simulink model "TopLevelModel"  (R2023a)
settings: Solver=VariableStepAuto  StartTime=0.0  StopTime=inf  RelTol=1e-3
values from neighbouring files (symbols this model uses):
  b = 40.6518    [TopLevelModelParameters.m]
  B1 = 0.0042    [TopLevelModelParameters.m]
  B2 = 0.0084    [TopLevelModelParameters.m]
  J1 = 7e-5    (= 7e-05)    [TopLevelModelParameters.m]
  J2 = 8e-5    (= 8e-05)    [TopLevelModelParameters.m]
  k1 = 2.6552e5    (= 265520)    [TopLevelModelParameters.m]
  k2 = 2.6552e5    (= 265520)    [TopLevelModelParameters.m]
  k3 = 11.777e4    (= 117770)    [TopLevelModelParameters.m]
  Kb = 23e-3    (= 0.023)    [TopLevelModelParameters.m]
  Kt = 23e-3    (= 0.023)    [TopLevelModelParameters.m]
  L = 0.1    [TopLevelModelParameters.m]
  m = 2    [TopLevelModelParameters.m]
  R = 0.71    [TopLevelModelParameters.m]
  r = 0.0194    [TopLevelModelParameters.m]
undefined symbols (not defined in the file or in its folder): J, Kd, Ke
libraries: fl_lib x40, fl_ps_legacy_lib x16, nesl_utility x12, slpidlib x10, SignalEditorBlockLib x4, ee_lib x4, simulink x2
(part 2 of 3)

== system TopLevelModel/Belt7 ==
  V1 : Inport
  Constant3 : Constant  Commented=on  Value=0.2
  Constant4 : Constant  Commented=on  Value=0
  PID Controller1 : slpidlib/PID Controller  Commented=on  Controller=PID  Form=Parallel  TimeDomain=Continuous-time  UseExternalTs=off  SampleTime=-1  IntegratorMethod=Forward Euler  FilterMethod=Forward Euler  ControllerParametersSource=internal  P=29.8496571480823  I=152.933850283855  UseKiTs=off  D=-0.451147774638306  N=4.48716691500189  UseFilter=on  TunerSelectOption=Transfer Function Based (PID Tuner App)  InitialConditionSource=internal  InitialConditionForIntegrator=0  InitialConditionForFilter=0  DifferentiatorICPrevScaledInput=0  ExternalReset=none  TrackingMode=off  Kt=1  LimitOutput=off  SatLimitsSource=internal  UpperSaturationLimit=inf  LowerSaturationLimit=-inf  LinearizeAsGain=on  AntiWindupMode=none  Kb=1  LimitIntegrator=off  UpperIntegratorSaturationLimit=inf  LowerIntegratorSaturationLimit=-inf  POutMin=[]  POutMax=[]  IOutMin=[]  IOutMax=[]  DOutMin=[]  DOutMax=[]  NOutMin=[]  NOutMax=[]  SumOutMin=[]  SumOutMax=[]  SaturationOutMin=[]  SaturationOutMax=[]  PParamMin=[]  PParamMax=[]  IParamMin=[]  IParamMax=[]  DParamMin=[]  DParamMax=[]  NParamMin=[]  NParamMax=[]  KbParamMin=[]  KbParamMax=[]  KtParamMin=[]  KtParamMax=[]  KbOutMin=[]  KbOutMax=[]  KtOutMin=[]  KtOutMax=[]  IntegratorOutMin=[]  IntegratorOutMax=[]  FilterOutMin=[]  FilterOutMax=[]  SumI1OutMin=[]  SumI1OutMax=[]  SumI2OutMin=[]  SumI2OutMax=[]  SumI3OutMin=[]  SumI3OutMax=[]  SumI4OutMin=[]  SumI4OutMax=[]  SumDOutMin=[]  SumDOutMax=[]  DifferentiatorOutMin=[]  DifferentiatorOutMax=[]  FilterDiffOutCoefMin=[]  FilterDiffOutCoefMax=[]  ReciprocalOutMin=[]  ReciprocalOutMax=[]  SumDenOutMin=[]  SumDenOutMax=[]  SumNumOutMin=[]  SumNumOutMax=[]  DivideOutMin=[]  DivideOutMax=[]  UdiffTsProdOutMin=[]  UdiffTsProdOutMax=[]  NTsProdOutMin=[]  NTsProdOutMax=[]  UintegralTsProdOutMin=[]  UintegralTsProdOutMax=[]  UngainTsProdOutMin=[]  UngainTsProdOutMax=[]  ClampingZeroOutDataTypeStr=Inherit: Inherit via back propagation  ClampingZeroOutMin=[]  ClampingZeroOutMax=[]  FilterDenConstantOutDataTypeStr=Inherit: Inherit via back propagation  FilterDenConstantOutMin=[]  FilterDenConstantOutMax=[]  PCopyOutDataTypeStr=Inherit: Inherit via back propagation  PCopyOutMin=[]  PCopyOutMax=[]  NCopyOutDataTypeStr=Inherit: Inherit via back propagation  NCopyOutMin=[]  NCopyOutMax=[]  IntegratorContinuousStateAttributes=''  IntegratorStateMustResolveToSignalObject=off  IntegratorRTWStateStorageClass=Auto  FilterContinuousStateAttributes=''  FilterStateMustResolveToSignalObject=off  FilterRTWStateStorageClass=Auto  ParallelPVariant=InternalParameters  IdealPVariant=Disabled  IVariant=InternalParameters  DVariant=InternalParameters  IntegratorVariant=Continuous  SatVariant=Disabled  AWVariant=Passthrough  PCopyVariant=Disabled  TRVariant=Disabled  FdbkBlocksVariant=Forward  IdealPFdbkVariant=Disabled  SatFdbkVariant=Disabled  DerivativeFilterVariant=ContFilter  NVariant=InternalParameters  NCopyVariant=Disabled  FilterICVariant=InternalICsFilter  IntegratorICVariant=InternalICs  ExternalResetVariant=Disabled  TRSumVariant=Passthrough  SumFdbkVariant=Disabled  SumVariant=Sum_PID  TsampFilterVariant=InternalTs  TsampNgainVariant=Passthrough  TsampIntegralVariant=Disabled_SignalSpec  ExternalSaturationOutDataTypeStr=Inherit: Same as second input
  Subsystem2 : Subsystem  Commented=on
  Sum1 : Sum  Commented=on  Inputs=|+-
  Switch1 : Switch  Commented=on  Criteria=u2 ~= 0  Threshold=1  SaturateOnIntegerOverflow=off  InputSameDT=off
  drive pulley velocity : Outport
  load velocity : Outport  Port=2
  load position : Outport  Port=3
  driven pulley Velocity : Outport  Port=4
  wires:
  Switch1/1 -> Sum1/1
  Sum1/1 -> PID Controller1/1
  V1/1 -> Switch1/2
  Subsystem2/2(load velocity) -> load velocity/1, Sum1/2  "Velocity"
  Constant3/1 -> Switch1/1
  Constant4/1 -> Switch1/3
  PID Controller1/1 -> Subsystem2/1(Voltage)
  Subsystem2/3(load position) -> load position/1
  Subsystem2/4(driven pulley Velocity) -> driven pulley Velocity/1
  Subsystem2/1(drive pulley velocity) -> drive pulley velocity/1

== system TopLevelModel/Belt8 ==
  V1 : Inport
  Constant3 : Constant  Commented=on  Value=0.2
  Constant4 : Constant  Commented=on  Value=0
  PID Controller1 : slpidlib/PID Controller  Commented=on  Controller=PID  Form=Parallel  TimeDomain=Continuous-time  UseExternalTs=off  SampleTime=-1  IntegratorMethod=Forward Euler  FilterMethod=Forward Euler  ControllerParametersSource=internal  P=29.8496571480823  I=152.933850283855  UseKiTs=off  D=-0.451147774638306  N=4.48716691500189  UseFilter=on  TunerSelectOption=Transfer Function Based (PID Tuner App)  InitialConditionSource=internal  InitialConditionForIntegrator=0  InitialConditionForFilter=0  DifferentiatorICPrevScaledInput=0  ExternalReset=none  TrackingMode=off  Kt=1  LimitOutput=off  SatLimitsSource=internal  UpperSaturationLimit=inf  LowerSaturationLimit=-inf  LinearizeAsGain=on  AntiWindupMode=none  Kb=1  LimitIntegrator=off  UpperIntegratorSaturationLimit=inf  LowerIntegratorSaturationLimit=-inf  POutMin=[]  POutMax=[]  IOutMin=[]  IOutMax=[]  DOutMin=[]  DOutMax=[]  NOutMin=[]  NOutMax=[]  SumOutMin=[]  SumOutMax=[]  SaturationOutMin=[]  SaturationOutMax=[]  PParamMin=[]  PParamMax=[]  IParamMin=[]  IParamMax=[]  DParamMin=[]  DParamMax=[]  NParamMin=[]  NParamMax=[]  KbParamMin=[]  KbParamMax=[]  KtParamMin=[]  KtParamMax=[]  KbOutMin=[]  KbOutMax=[]  KtOutMin=[]  KtOutMax=[]  IntegratorOutMin=[]  IntegratorOutMax=[]  FilterOutMin=[]  FilterOutMax=[]  SumI1OutMin=[]  SumI1OutMax=[]  SumI2OutMin=[]  SumI2OutMax=[]  SumI3OutMin=[]  SumI3OutMax=[]  SumI4OutMin=[]  SumI4OutMax=[]  SumDOutMin=[]  SumDOutMax=[]  DifferentiatorOutMin=[]  DifferentiatorOutMax=[]  FilterDiffOutCoefMin=[]  FilterDiffOutCoefMax=[]  ReciprocalOutMin=[]  ReciprocalOutMax=[]  SumDenOutMin=[]  SumDenOutMax=[]  SumNumOutMin=[]  SumNumOutMax=[]  DivideOutMin=[]  DivideOutMax=[]  UdiffTsProdOutMin=[]  UdiffTsProdOutMax=[]  NTsProdOutMin=[]  NTsProdOutMax=[]  UintegralTsProdOutMin=[]  UintegralTsProdOutMax=[]  UngainTsProdOutMin=[]  UngainTsProdOutMax=[]  ClampingZeroOutDataTypeStr=Inherit: Inherit via back propagation  ClampingZeroOutMin=[]  ClampingZeroOutMax=[]  FilterDenConstantOutDataTypeStr=Inherit: Inherit via back propagation  FilterDenConstantOutMin=[]  FilterDenConstantOutMax=[]  PCopyOutDataTypeStr=Inherit: Inherit via back propagation  PCopyOutMin=[]  PCopyOutMax=[]  NCopyOutDataTypeStr=Inherit: Inherit via back propagation  NCopyOutMin=[]  NCopyOutMax=[]  IntegratorContinuousStateAttributes=''  IntegratorStateMustResolveToSignalObject=off  IntegratorRTWStateStorageClass=Auto  FilterContinuousStateAttributes=''  FilterStateMustResolveToSignalObject=off  FilterRTWStateStorageClass=Auto  ParallelPVariant=InternalParameters  IdealPVariant=Disabled  IVariant=InternalParameters  DVariant=InternalParameters  IntegratorVariant=Continuous  SatVariant=Disabled  AWVariant=Passthrough  PCopyVariant=Disabled  TRVariant=Disabled  FdbkBlocksVariant=Forward  IdealPFdbkVariant=Disabled  SatFdbkVariant=Disabled  DerivativeFilterVariant=ContFilter  NVariant=InternalParameters  NCopyVariant=Disabled  FilterICVariant=InternalICsFilter  IntegratorICVariant=InternalICs  ExternalResetVariant=Disabled  TRSumVariant=Passthrough  SumFdbkVariant=Disabled  SumVariant=Sum_PID  TsampFilterVariant=InternalTs  TsampNgainVariant=Passthrough  TsampIntegralVariant=Disabled_SignalSpec  ExternalSaturationOutDataTypeStr=Inherit: Same as second input
  Subsystem2 : Subsystem  Commented=on
  Sum1 : Sum  Commented=on  Inputs=|+-
  Switch1 : Switch  Commented=on  Criteria=u2 ~= 0  Threshold=1  SaturateOnIntegerOverflow=off  InputSameDT=off
  drive pulley velocity : Outport
  load velocity : Outport  Port=2
  load position : Outport  Port=3
  driven pulley Velocity : Outport  Port=4
  wires:
  Switch1/1 -> Sum1/1
  Sum1/1 -> PID Controller1/1
  V1/1 -> Switch1/2
  Subsystem2/2(load velocity) -> load velocity/1, Sum1/2  "Velocity"
  Constant3/1 -> Switch1/1
  Constant4/1 -> Switch1/3
  PID Controller1/1 -> Subsystem2/1(Voltage)
  Subsystem2/3(load position) -> load position/1
  Subsystem2/4(driven pulley Velocity) -> driven pulley Velocity/1
  Subsystem2/1(drive pulley velocity) -> drive pulley velocity/1

== system TopLevelModel/Belt9 ==
  V1 : Inport
  Constant3 : Constant  Commented=on  Value=0.2
  Constant4 : Constant  Commented=on  Value=0
  PID Controller1 : slpidlib/PID Controller  Commented=on  Controller=PID  Form=Parallel  TimeDomain=Continuous-time  UseExternalTs=off  SampleTime=-1  IntegratorMethod=Forward Euler  FilterMethod=Forward Euler  ControllerParametersSource=internal  P=29.8496571480823  I=152.933850283855  UseKiTs=off  D=-0.451147774638306  N=4.48716691500189  UseFilter=on  TunerSelectOption=Transfer Function Based (PID Tuner App)  InitialConditionSource=internal  InitialConditionForIntegrator=0  InitialConditionForFilter=0  DifferentiatorICPrevScaledInput=0  ExternalReset=none  TrackingMode=off  Kt=1  LimitOutput=off  SatLimitsSource=internal  UpperSaturationLimit=inf  LowerSaturationLimit=-inf  LinearizeAsGain=on  AntiWindupMode=none  Kb=1  LimitIntegrator=off  UpperIntegratorSaturationLimit=inf  LowerIntegratorSaturationLimit=-inf  POutMin=[]  POutMax=[]  IOutMin=[]  IOutMax=[]  DOutMin=[]  DOutMax=[]  NOutMin=[]  NOutMax=[]  SumOutMin=[]  SumOutMax=[]  SaturationOutMin=[]  SaturationOutMax=[]  PParamMin=[]  PParamMax=[]  IParamMin=[]  IParamMax=[]  DParamMin=[]  DParamMax=[]  NParamMin=[]  NParamMax=[]  KbParamMin=[]  KbParamMax=[]  KtParamMin=[]  KtParamMax=[]  KbOutMin=[]  KbOutMax=[]  KtOutMin=[]  KtOutMax=[]  IntegratorOutMin=[]  IntegratorOutMax=[]  FilterOutMin=[]  FilterOutMax=[]  SumI1OutMin=[]  SumI1OutMax=[]  SumI2OutMin=[]  SumI2OutMax=[]  SumI3OutMin=[]  SumI3OutMax=[]  SumI4OutMin=[]  SumI4OutMax=[]  SumDOutMin=[]  SumDOutMax=[]  DifferentiatorOutMin=[]  DifferentiatorOutMax=[]  FilterDiffOutCoefMin=[]  FilterDiffOutCoefMax=[]  ReciprocalOutMin=[]  ReciprocalOutMax=[]  SumDenOutMin=[]  SumDenOutMax=[]  SumNumOutMin=[]  SumNumOutMax=[]  DivideOutMin=[]  DivideOutMax=[]  UdiffTsProdOutMin=[]  UdiffTsProdOutMax=[]  NTsProdOutMin=[]  NTsProdOutMax=[]  UintegralTsProdOutMin=[]  UintegralTsProdOutMax=[]  UngainTsProdOutMin=[]  UngainTsProdOutMax=[]  ClampingZeroOutDataTypeStr=Inherit: Inherit via back propagation  ClampingZeroOutMin=[]  ClampingZeroOutMax=[]  FilterDenConstantOutDataTypeStr=Inherit: Inherit via back propagation  FilterDenConstantOutMin=[]  FilterDenConstantOutMax=[]  PCopyOutDataTypeStr=Inherit: Inherit via back propagation  PCopyOutMin=[]  PCopyOutMax=[]  NCopyOutDataTypeStr=Inherit: Inherit via back propagation  NCopyOutMin=[]  NCopyOutMax=[]  IntegratorContinuousStateAttributes=''  IntegratorStateMustResolveToSignalObject=off  IntegratorRTWStateStorageClass=Auto  FilterContinuousStateAttributes=''  FilterStateMustResolveToSignalObject=off  FilterRTWStateStorageClass=Auto  ParallelPVariant=InternalParameters  IdealPVariant=Disabled  IVariant=InternalParameters  DVariant=InternalParameters  IntegratorVariant=Continuous  SatVariant=Disabled  AWVariant=Passthrough  PCopyVariant=Disabled  TRVariant=Disabled  FdbkBlocksVariant=Forward  IdealPFdbkVariant=Disabled  SatFdbkVariant=Disabled  DerivativeFilterVariant=ContFilter  NVariant=InternalParameters  NCopyVariant=Disabled  FilterICVariant=InternalICsFilter  IntegratorICVariant=InternalICs  ExternalResetVariant=Disabled  TRSumVariant=Passthrough  SumFdbkVariant=Disabled  SumVariant=Sum_PID  TsampFilterVariant=InternalTs  TsampNgainVariant=Passthrough  TsampIntegralVariant=Disabled_SignalSpec  ExternalSaturationOutDataTypeStr=Inherit: Same as second input
  Subsystem2 : Subsystem  Commented=on
  Sum1 : Sum  Commented=on  Inputs=|+-
  Switch1 : Switch  Commented=on  Criteria=u2 ~= 0  Threshold=1  SaturateOnIntegerOverflow=off  InputSameDT=off
  drive pulley velocity : Outport
  load velocity : Outport  Port=2
  load position : Outport  Port=3
  driven pulley Velocity : Outport  Port=4
  wires:
  Switch1/1 -> Sum1/1
  Sum1/1 -> PID Controller1/1
  V1/1 -> Switch1/2
  Subsystem2/2(load velocity) -> load velocity/1, Sum1/2  "Velocity"
  Constant3/1 -> Switch1/1
  Constant4/1 -> Switch1/3
  PID Controller1/1 -> Subsystem2/1(Voltage)
  Subsystem2/3(load position) -> load position/1
  Subsystem2/4(driven pulley Velocity) -> driven pulley Velocity/1
  Subsystem2/1(drive pulley velocity) -> drive pulley velocity/1

== system TopLevelModel/Controller ==
  Ref : Inport
  Position : Subsystem  VariantControl=Position
  Speed : Subsystem  VariantControl=Speed
  PWM : PMIOPort  Side=Right
  0v : PMIOPort  Port=2  Side=Right
  REV : PMIOPort  Port=3  Side=Right

== system TopLevelModel/Controller1 ==
  Ref : Inport
  Position : Subsystem  VariantControl=Position
  Speed : Subsystem  VariantControl=Speed
  PWM : PMIOPort  Side=Right
  0v : PMIOPort  Port=2  Side=Right
  REV : PMIOPort  Port=3  Side=Right

== system TopLevelModel/DC Motor10 ==
  note: Armature Controlled DC Motor
      |
      | $E_a = R_a \cdot I_a + L_a \cdot \frac{di_a}{dt} + K_b \cdot \frac{d\theta}{dt}$
      | $T_{m} = K_{t} \cdot I_{a}$
  Voltage : Inport
  Velocity : Inport  Port=2
  Constant1 : Constant  Value=R
  Gain1 : Gain  Gain=Kb
  Gain2 : Gain  Gain=1/L
  Gain3 : Gain  Gain=Kt
  Integrator : Integrator
  Product : Product
  Subtract : Sum  Inputs=+--
  Tourque : Outport
  wires:
  Voltage/1 -> Subtract/1
  Integrator/1 -> Product/1, Gain3/1  "i"
  Gain3/1 -> Tourque/1
  Gain1/1 -> Subtract/2
  Velocity/1 -> Gain1/1
  Constant1/1 -> Product/2
  Product/1 -> Subtract/3
  Gain2/1 -> Integrator/1  "i_dot"
  Subtract/1 -> Gain2/1

== system TopLevelModel/Sensing Angle ==
  MRRef : fl_lib/Mechanical/Rotational Elements/Mechanical Rotational Reference
  Motion Sensor : fl_lib/Mechanical/Mechanical Sensors/Ideal Rotational Motion Sensor  reference=foundation.enum.MeasurementReference.difference  acceleration_port=false  velocity_port=true  position_port=true  wrap_angle=simscape.enum.onoff.off  offset=0 rad
  deg : nesl_utility/PS-Simulink Converter  PhysicalDomain=network_engine_domain  SubClassName=ps_output  LeftPortType=input  RightPortType=output  PseudoPeriodic=off  Frequencies=[]  VectorFormat=1-D array  Unit=deg  AffineConversion=off
  R : PMIOPort  Side=Left
  theta : Outport  VectorParamsAs1DForOutWhenUnconnected=off
  wires:
  deg/1 -> theta/1
  connections:
  R/RConn1 -- Motion Sensor/LConn1
  Motion Sensor/RConn3 -- deg/LConn1
  MRRef/LConn1 -- Motion Sensor/RConn1

== system TopLevelModel/Sensing Angle1 ==
  MRRef : fl_lib/Mechanical/Rotational Elements/Mechanical Rotational Reference
  Motion Sensor : fl_lib/Mechanical/Mechanical Sensors/Ideal Rotational Motion Sensor  reference=foundation.enum.MeasurementReference.difference  acceleration_port=false  velocity_port=true  position_port=true  wrap_angle=simscape.enum.onoff.off  offset=0 rad
  deg : nesl_utility/PS-Simulink Converter  PhysicalDomain=network_engine_domain  SubClassName=ps_output  LeftPortType=input  RightPortType=output  PseudoPeriodic=off  Frequencies=[]  VectorFormat=1-D array  Unit=deg  AffineConversion=off
  R : PMIOPort  Side=Left
  theta : Outport  VectorParamsAs1DForOutWhenUnconnected=off
  wires:
  deg/1 -> theta/1
  connections:
  R/RConn1 -- Motion Sensor/LConn1
  Motion Sensor/RConn3 -- deg/LConn1
  MRRef/LConn1 -- Motion Sensor/RConn1

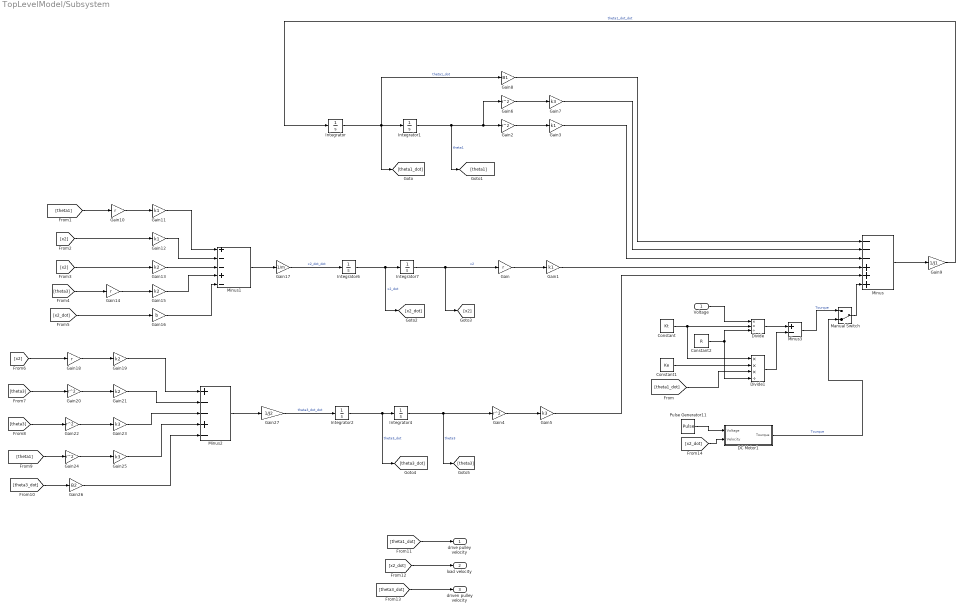
== system TopLevelModel/Subsystem ==
  Voltage : Inport
  Constant : Constant  Value=Kt
  Constant1 : Constant  Value=Ke
  Constant2 : Constant  Value=R
  DC Motor1 : Subsystem
  Divide : Product  Inputs=**/
  Divide1 : Product  Inputs=***/
  Gain{,10,14,18} (4 alike) : Gain  Gain=r
  Gain{1,3,11..12} (4 alike) : Gain  Gain=k1
  Gain{13,15,19,21} (4 alike) : Gain  Gain=k2
  Gain16 : Gain  Gain=b
  Gain17 : Gain  Gain=1/m
  Gain{2,4,6,20,22,24} (6 alike) : Gain  Gain=r^2
  Gain{5,7,23,25} (4 alike) : Gain  Gain=k3
  Gain26 : Gain  Gain=B2
  Gain27 : Gain  Gain=1/J2
  Gain8 : Gain  Gain=B1
  Gain9 : Gain  Gain=1/J1
  Integrator{,1..2,4,6..7} (6 alike) : Integrator
  Manual Switch : ManualSwitch  CurrentSetting=0
  Minus : Sum  Inputs=---+++
  Minus1 : Sum  Inputs=+--+-
  Minus2 : Sum  Inputs=+--+-
  Minus3 : Sum  Inputs=+-
  Pulse Generator11 : DiscretePulseGenerator  PulseType=Time based  Amplitude=12  Period=11  PulseWidth=50  PhaseDelay=2
  drive pulley velocity : Outport
  load velocity : Outport  Port=2
  driven pulley velocity : Outport  Port=3
  wires:
  Gain23/1 -> Minus2/3
  Gain4/1 -> Gain5/1
  [theta1] -> Gain24/1
  Gain11/1 -> Minus1/1
  [theta3_dot] -> Gain26/1
  Gain26/1 -> Minus2/5
  Gain22/1 -> Gain23/1
  Gain19/1 -> Minus2/1
  Gain21/1 -> Minus2/2
  Integrator/1 -> Integrator1/1, [theta1_dot], Gain8/1  "theta1_dot"
  Integrator1/1 -> Gain6/1, Gain2/1, [theta1]  "theta1"
  Integrator6/1 -> Integrator7/1, [x2_dot]  "x2_dot"
  Gain3/1 -> Minus/3
  Gain18/1 -> Gain19/1
  Gain1/1 -> Minus/4
  Gain2/1 -> Gain3/1
  Integrator2/1 -> [theta3_dot], Integrator4/1  "theta3_dot"
  Integrator4/1 -> Gain4/1, [theta3]  "theta3"
  [x2] -> Gain12/1
  Gain/1 -> Gain1/1
  Gain10/1 -> Gain11/1
  [theta1_dot] -> Divide1/3
  Gain24/1 -> Gain25/1
  Gain13/1 -> Minus1/3
  [theta3] -> Gain20/1
  [theta3] -> Gain14/1
  Gain15/1 -> Minus1/4
  Gain6/1 -> Gain7/1
  [theta3] -> Gain22/1
  Gain5/1 -> Minus/5
  [theta1] -> Gain10/1
  [x2] -> Gain18/1
  Minus2/1 -> Gain27/1
  Minus1/1 -> Gain17/1
  Minus/1 -> Gain9/1
  Gain7/1 -> Minus/2
  Integrator7/1 -> Gain/1, [x2]  "x2"
  Gain16/1 -> Minus1/5
  Gain8/1 -> Minus/1
  Gain17/1 -> Integrator6/1  "x2_dot_dot"
  Gain14/1 -> Gain15/1
  Gain20/1 -> Gain21/1
  Gain9/1 -> Integrator/1  "theta1_dot_dot"
  Gain12/1 -> Minus1/2
  Gain25/1 -> Minus2/4
  [x2] -> Gain13/1
  Minus3/1 -> Manual Switch/1  "Tourque"
  [x2_dot] -> Gain16/1
  [theta1_dot] -> drive pulley velocity/1
  [x2_dot] -> load velocity/1
  [theta3_dot] -> driven pulley velocity/1
  Gain27/1 -> Integrator2/1  "theta3_dot_dot"
  Voltage/1 -> Divide/1
  Constant/1 -> Divide/2, Divide1/1
  Constant2/1 -> Divide1/4, Divide/3
  Divide/1 -> Minus3/1
  Constant1/1 -> Divide1/2
  Divide1/1 -> Minus3/2
  Manual Switch/1 -> Minus/6
  DC Motor1/1(Tourque) -> Manual Switch/2  "Tourque"
  Pulse Generator11/1 -> DC Motor1/1(Voltage)
  [x2_dot] -> DC Motor1/2(Velocity)

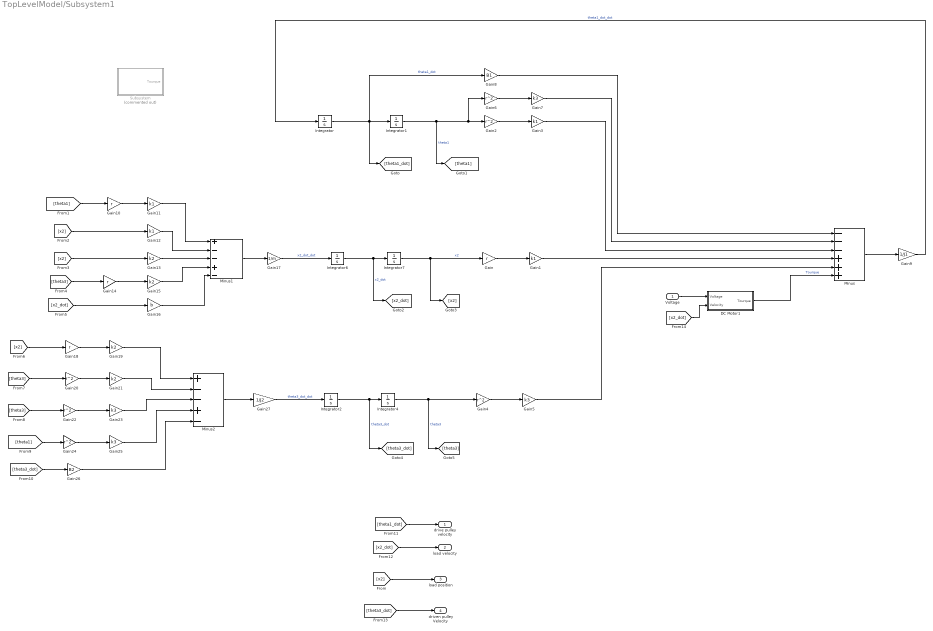
== system TopLevelModel/Subsystem1 ==
  Voltage : Inport
  DC Motor1 : Subsystem
  Gain{,10,14,18} (4 alike) : Gain  Gain=r
  Gain{1,3,11..12} (4 alike) : Gain  Gain=k1
  Gain{13,15,19,21} (4 alike) : Gain  Gain=k2
  Gain16 : Gain  Gain=b
  Gain17 : Gain  Gain=1/m
  Gain{2,4,6,20,22,24} (6 alike) : Gain  Gain=r^2
  Gain{5,7,23,25} (4 alike) : Gain  Gain=k3
  Gain26 : Gain  Gain=B2
  Gain27 : Gain  Gain=1/J2
  Gain8 : Gain  Gain=B1
  Gain9 : Gain  Gain=1/J1
  Integrator{,1..2,4,6..7} (6 alike) : Integrator
  Minus : Sum  Inputs=---+++
  Minus1 : Sum  Inputs=+--+-
  Minus2 : Sum  Inputs=+--+-
  Subsystem : Subsystem  Commented=on
  drive pulley velocity : Outport
  load velocity : Outport  Port=2
  load position : Outport  Port=3
  driven pulley Velocity : Outport  Port=4
  wires:
  Gain23/1 -> Minus2/3
  Gain4/1 -> Gain5/1
  [theta1] -> Gain24/1
  Gain11/1 -> Minus1/1
  [theta3_dot] -> Gain26/1
  Gain26/1 -> Minus2/5
  Gain22/1 -> Gain23/1
  Gain19/1 -> Minus2/1
  Gain21/1 -> Minus2/2
  Integrator/1 -> Integrator1/1, [theta1_dot], Gain8/1  "theta1_dot"
  Integrator1/1 -> Gain6/1, Gain2/1, [theta1]  "theta1"
  Integrator6/1 -> Integrator7/1, [x2_dot]  "x2_dot"
  Gain3/1 -> Minus/3
  Gain18/1 -> Gain19/1
  Gain1/1 -> Minus/4
  Gain2/1 -> Gain3/1
  Integrator2/1 -> [theta3_dot], Integrator4/1  "theta3_dot"
  Integrator4/1 -> Gain4/1, [theta3]  "theta3"
  [x2] -> Gain12/1
  Gain/1 -> Gain1/1
  Gain10/1 -> Gain11/1
  Gain24/1 -> Gain25/1
  Gain13/1 -> Minus1/3
  [theta3] -> Gain20/1
  [theta3] -> Gain14/1
  Gain15/1 -> Minus1/4
  Gain6/1 -> Gain7/1
  [theta3] -> Gain22/1
  Gain5/1 -> Minus/5
  [theta1] -> Gain10/1
  [x2] -> Gain18/1
  Minus2/1 -> Gain27/1
  Minus1/1 -> Gain17/1
  Minus/1 -> Gain9/1
  Gain7/1 -> Minus/2
  Integrator7/1 -> Gain/1, [x2]  "x2"
  Gain16/1 -> Minus1/5
  Gain8/1 -> Minus/1
  Gain17/1 -> Integrator6/1  "x2_dot_dot"
  Gain14/1 -> Gain15/1
  Gain20/1 -> Gain21/1
  Gain9/1 -> Integrator/1  "theta1_dot_dot"
  Gain12/1 -> Minus1/2
  Gain25/1 -> Minus2/4
  [x2] -> Gain13/1
  [x2_dot] -> Gain16/1
  [theta1_dot] -> drive pulley velocity/1
  [x2_dot] -> load velocity/1
  Gain27/1 -> Integrator2/1  "theta3_dot_dot"
  DC Motor1/1(Tourque) -> Minus/6  "Tourque"
  [x2_dot] -> DC Motor1/2(Velocity)
  Voltage/1 -> DC Motor1/1(Voltage)
  [x2] -> load position/1
  [theta3_dot] -> driven pulley Velocity/1

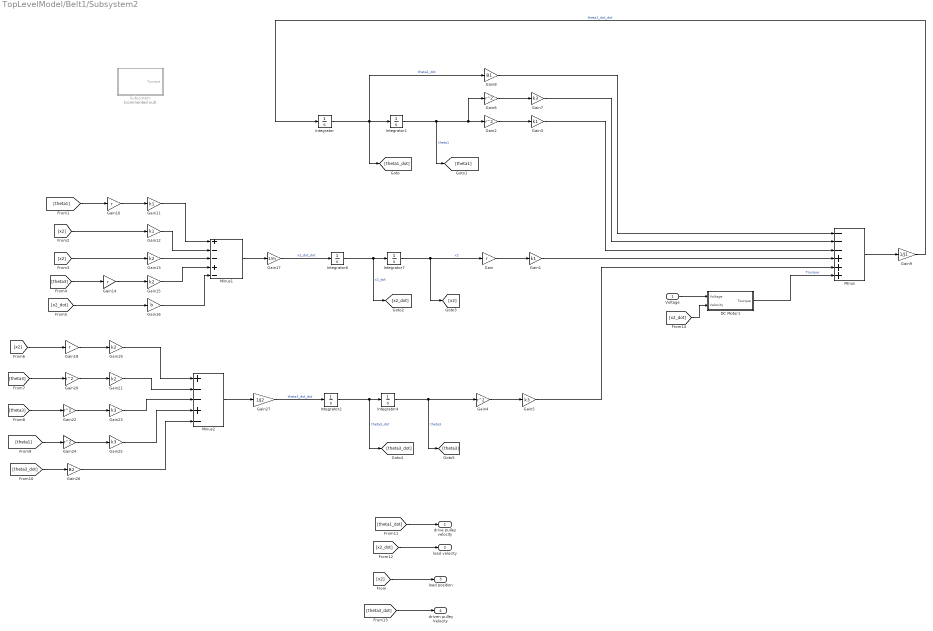
== system TopLevelModel/Belt1/Subsystem2 ==
  Voltage : Inport
  DC Motor1 : Subsystem
  Gain{,10,14,18} (4 alike) : Gain  Gain=r
  Gain{1,3,11..12} (4 alike) : Gain  Gain=k1
  Gain{13,15,19,21} (4 alike) : Gain  Gain=k2
  Gain16 : Gain  Gain=b
  Gain17 : Gain  Gain=1/m
  Gain{2,4,6,20,22,24} (6 alike) : Gain  Gain=r^2
  Gain{5,7,23,25} (4 alike) : Gain  Gain=k3
  Gain26 : Gain  Gain=B2
  Gain27 : Gain  Gain=1/J2
  Gain8 : Gain  Gain=B1
  Gain9 : Gain  Gain=1/J1
  Integrator{,1..2,4,6..7} (6 alike) : Integrator
  Minus : Sum  Inputs=---+++
  Minus1 : Sum  Inputs=+--+-
  Minus2 : Sum  Inputs=+--+-
  Subsystem : Subsystem  Commented=on
  drive pulley velocity : Outport
  load velocity : Outport  Port=2
  load position : Outport  Port=3
  driven pulley Velocity : Outport  Port=4
  wires:
  Gain23/1 -> Minus2/3
  Gain4/1 -> Gain5/1
  [theta1] -> Gain24/1
  Gain11/1 -> Minus1/1
  [theta3_dot] -> Gain26/1
  Gain26/1 -> Minus2/5
  Gain22/1 -> Gain23/1
  Gain19/1 -> Minus2/1
  Gain21/1 -> Minus2/2
  Integrator/1 -> Integrator1/1, [theta1_dot], Gain8/1  "theta1_dot"
  Integrator1/1 -> Gain6/1, Gain2/1, [theta1]  "theta1"
  Integrator6/1 -> Integrator7/1, [x2_dot]  "x2_dot"
  Gain3/1 -> Minus/3
  Gain18/1 -> Gain19/1
  Gain1/1 -> Minus/4
  Gain2/1 -> Gain3/1
  Integrator2/1 -> [theta3_dot], Integrator4/1  "theta3_dot"
  Integrator4/1 -> Gain4/1, [theta3]  "theta3"
  [x2] -> Gain12/1
  Gain/1 -> Gain1/1
  Gain10/1 -> Gain11/1
  Gain24/1 -> Gain25/1
  Gain13/1 -> Minus1/3
  [theta3] -> Gain20/1
  [theta3] -> Gain14/1
  Gain15/1 -> Minus1/4
  Gain6/1 -> Gain7/1
  [theta3] -> Gain22/1
  Gain5/1 -> Minus/5
  [theta1] -> Gain10/1
  [x2] -> Gain18/1
  Minus2/1 -> Gain27/1
  Minus1/1 -> Gain17/1
  Minus/1 -> Gain9/1
  Gain7/1 -> Minus/2
  Integrator7/1 -> Gain/1, [x2]  "x2"
  Gain16/1 -> Minus1/5
  Gain8/1 -> Minus/1
  Gain17/1 -> Integrator6/1  "x2_dot_dot"
  Gain14/1 -> Gain15/1
  Gain20/1 -> Gain21/1
  Gain9/1 -> Integrator/1  "theta1_dot_dot"
  Gain12/1 -> Minus1/2
  Gain25/1 -> Minus2/4
  [x2] -> Gain13/1
  [x2_dot] -> Gain16/1
  [theta1_dot] -> drive pulley velocity/1
  [x2_dot] -> load velocity/1
  Gain27/1 -> Integrator2/1  "theta3_dot_dot"
  DC Motor1/1(Tourque) -> Minus/6  "Tourque"
  [x2_dot] -> DC Motor1/2(Velocity)
  Voltage/1 -> DC Motor1/1(Voltage)
  [x2] -> load position/1
  [theta3_dot] -> driven pulley Velocity/1

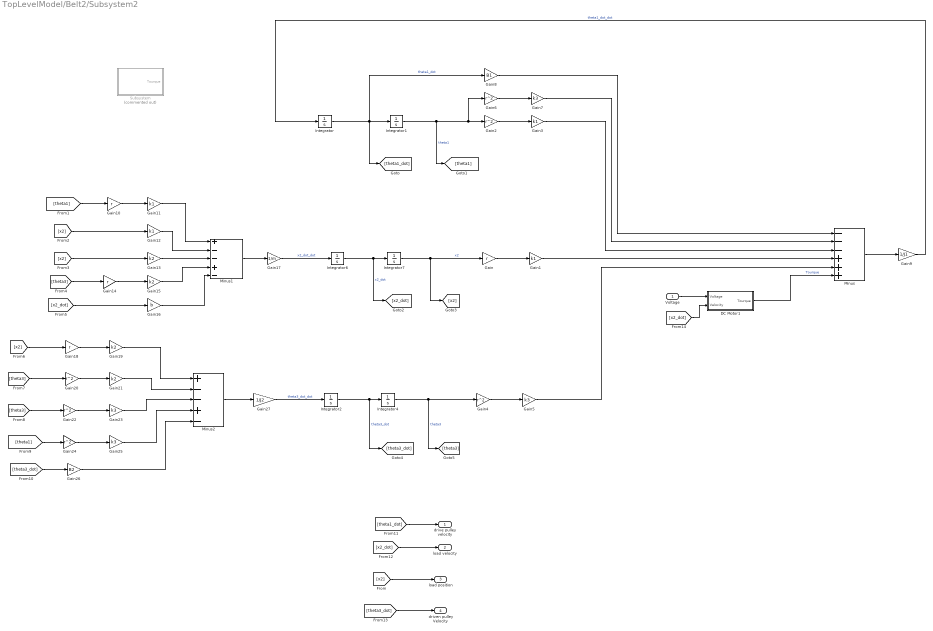
== system TopLevelModel/Belt2/Subsystem2 ==
  Voltage : Inport
  DC Motor1 : Subsystem
  Gain{,10,14,18} (4 alike) : Gain  Gain=r
  Gain{1,3,11..12} (4 alike) : Gain  Gain=k1
  Gain{13,15,19,21} (4 alike) : Gain  Gain=k2
  Gain16 : Gain  Gain=b
  Gain17 : Gain  Gain=1/m
  Gain{2,4,6,20,22,24} (6 alike) : Gain  Gain=r^2
  Gain{5,7,23,25} (4 alike) : Gain  Gain=k3
  Gain26 : Gain  Gain=B2
  Gain27 : Gain  Gain=1/J2
  Gain8 : Gain  Gain=B1
  Gain9 : Gain  Gain=1/J1
  Integrator{,1..2,4,6..7} (6 alike) : Integrator
  Minus : Sum  Inputs=---+++
  Minus1 : Sum  Inputs=+--+-
  Minus2 : Sum  Inputs=+--+-
  Subsystem : Subsystem  Commented=on
  drive pulley velocity : Outport
  load velocity : Outport  Port=2
  load position : Outport  Port=3
  driven pulley Velocity : Outport  Port=4
  wires:
  Gain23/1 -> Minus2/3
  Gain4/1 -> Gain5/1
  [theta1] -> Gain24/1
  Gain11/1 -> Minus1/1
  [theta3_dot] -> Gain26/1
  Gain26/1 -> Minus2/5
  Gain22/1 -> Gain23/1
  Gain19/1 -> Minus2/1
  Gain21/1 -> Minus2/2
  Integrator/1 -> Integrator1/1, [theta1_dot], Gain8/1  "theta1_dot"
  Integrator1/1 -> Gain6/1, Gain2/1, [theta1]  "theta1"
  Integrator6/1 -> Integrator7/1, [x2_dot]  "x2_dot"
  Gain3/1 -> Minus/3
  Gain18/1 -> Gain19/1
  Gain1/1 -> Minus/4
  Gain2/1 -> Gain3/1
  Integrator2/1 -> [theta3_dot], Integrator4/1  "theta3_dot"
  Integrator4/1 -> Gain4/1, [theta3]  "theta3"
  [x2] -> Gain12/1
  Gain/1 -> Gain1/1
  Gain10/1 -> Gain11/1
  Gain24/1 -> Gain25/1
  Gain13/1 -> Minus1/3
  [theta3] -> Gain20/1
  [theta3] -> Gain14/1
  Gain15/1 -> Minus1/4
  Gain6/1 -> Gain7/1
  [theta3] -> Gain22/1
  Gain5/1 -> Minus/5
  [theta1] -> Gain10/1
  [x2] -> Gain18/1
  Minus2/1 -> Gain27/1
  Minus1/1 -> Gain17/1
  Minus/1 -> Gain9/1
  Gain7/1 -> Minus/2
  Integrator7/1 -> Gain/1, [x2]  "x2"
  Gain16/1 -> Minus1/5
  Gain8/1 -> Minus/1
  Gain17/1 -> Integrator6/1  "x2_dot_dot"
  Gain14/1 -> Gain15/1
  Gain20/1 -> Gain21/1
  Gain9/1 -> Integrator/1  "theta1_dot_dot"
  Gain12/1 -> Minus1/2
  Gain25/1 -> Minus2/4
  [x2] -> Gain13/1
  [x2_dot] -> Gain16/1
  [theta1_dot] -> drive pulley velocity/1
  [x2_dot] -> load velocity/1
  Gain27/1 -> Integrator2/1  "theta3_dot_dot"
  DC Motor1/1(Tourque) -> Minus/6  "Tourque"
  [x2_dot] -> DC Motor1/2(Velocity)
  Voltage/1 -> DC Motor1/1(Voltage)
  [x2] -> load position/1
  [theta3_dot] -> driven pulley Velocity/1

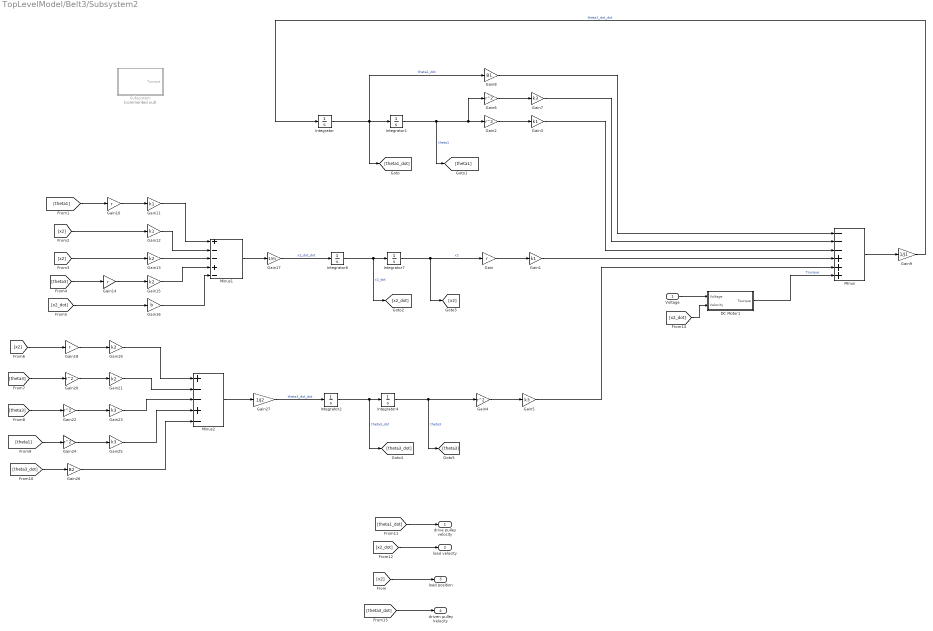
== system TopLevelModel/Belt3/Subsystem2 ==
  Voltage : Inport
  DC Motor1 : Subsystem
  Gain{,10,14,18} (4 alike) : Gain  Gain=r
  Gain{1,3,11..12} (4 alike) : Gain  Gain=k1
  Gain{13,15,19,21} (4 alike) : Gain  Gain=k2
  Gain16 : Gain  Gain=b
  Gain17 : Gain  Gain=1/m
  Gain{2,4,6,20,22,24} (6 alike) : Gain  Gain=r^2
  Gain{5,7,23,25} (4 alike) : Gain  Gain=k3
  Gain26 : Gain  Gain=B2
  Gain27 : Gain  Gain=1/J2
  Gain8 : Gain  Gain=B1
  Gain9 : Gain  Gain=1/J1
  Integrator{,1..2,4,6..7} (6 alike) : Integrator
  Minus : Sum  Inputs=---+++
  Minus1 : Sum  Inputs=+--+-
  Minus2 : Sum  Inputs=+--+-
  Subsystem : Subsystem  Commented=on
  drive pulley velocity : Outport
  load velocity : Outport  Port=2
  load position : Outport  Port=3
  driven pulley Velocity : Outport  Port=4
  wires:
  Gain23/1 -> Minus2/3
  Gain4/1 -> Gain5/1
  [theta1] -> Gain24/1
  Gain11/1 -> Minus1/1
  [theta3_dot] -> Gain26/1
  Gain26/1 -> Minus2/5
  Gain22/1 -> Gain23/1
  Gain19/1 -> Minus2/1
  Gain21/1 -> Minus2/2
  Integrator/1 -> Integrator1/1, [theta1_dot], Gain8/1  "theta1_dot"
  Integrator1/1 -> Gain6/1, Gain2/1, [theta1]  "theta1"
  Integrator6/1 -> Integrator7/1, [x2_dot]  "x2_dot"
  Gain3/1 -> Minus/3
  Gain18/1 -> Gain19/1
  Gain1/1 -> Minus/4
  Gain2/1 -> Gain3/1
  Integrator2/1 -> [theta3_dot], Integrator4/1  "theta3_dot"
  Integrator4/1 -> Gain4/1, [theta3]  "theta3"
  [x2] -> Gain12/1
  Gain/1 -> Gain1/1
  Gain10/1 -> Gain11/1
  Gain24/1 -> Gain25/1
  Gain13/1 -> Minus1/3
  [theta3] -> Gain20/1
  [theta3] -> Gain14/1
  Gain15/1 -> Minus1/4
  Gain6/1 -> Gain7/1
  [theta3] -> Gain22/1
  Gain5/1 -> Minus/5
  [theta1] -> Gain10/1
  [x2] -> Gain18/1
  Minus2/1 -> Gain27/1
  Minus1/1 -> Gain17/1
  Minus/1 -> Gain9/1
  Gain7/1 -> Minus/2
  Integrator7/1 -> Gain/1, [x2]  "x2"
  Gain16/1 -> Minus1/5
  Gain8/1 -> Minus/1
  Gain17/1 -> Integrator6/1  "x2_dot_dot"
  Gain14/1 -> Gain15/1
  Gain20/1 -> Gain21/1
  Gain9/1 -> Integrator/1  "theta1_dot_dot"
  Gain12/1 -> Minus1/2
  Gain25/1 -> Minus2/4
  [x2] -> Gain13/1
  [x2_dot] -> Gain16/1
  [theta1_dot] -> drive pulley velocity/1
  [x2_dot] -> load velocity/1
  Gain27/1 -> Integrator2/1  "theta3_dot_dot"
  DC Motor1/1(Tourque) -> Minus/6  "Tourque"
  [x2_dot] -> DC Motor1/2(Velocity)
  Voltage/1 -> DC Motor1/1(Voltage)
  [x2] -> load position/1
  [theta3_dot] -> driven pulley Velocity/1

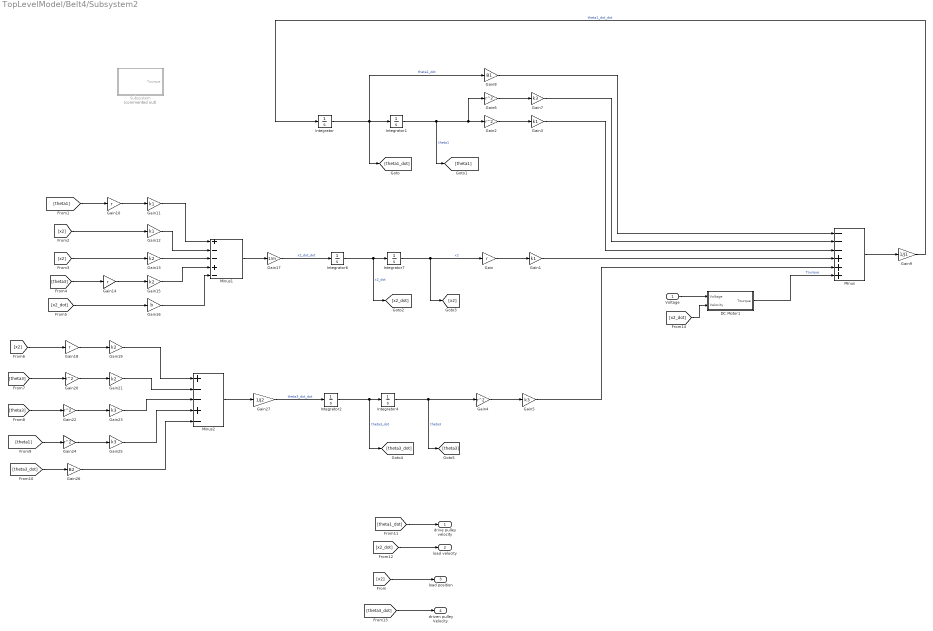
== system TopLevelModel/Belt4/Subsystem2 ==
  Voltage : Inport
  DC Motor1 : Subsystem
  Gain{,10,14,18} (4 alike) : Gain  Gain=r
  Gain{1,3,11..12} (4 alike) : Gain  Gain=k1
  Gain{13,15,19,21} (4 alike) : Gain  Gain=k2
  Gain16 : Gain  Gain=b
  Gain17 : Gain  Gain=1/m
  Gain{2,4,6,20,22,24} (6 alike) : Gain  Gain=r^2
  Gain{5,7,23,25} (4 alike) : Gain  Gain=k3
  Gain26 : Gain  Gain=B2
  Gain27 : Gain  Gain=1/J2
  Gain8 : Gain  Gain=B1
  Gain9 : Gain  Gain=1/J1
  Integrator{,1..2,4,6..7} (6 alike) : Integrator
  Minus : Sum  Inputs=---+++
  Minus1 : Sum  Inputs=+--+-
  Minus2 : Sum  Inputs=+--+-
  Subsystem : Subsystem  Commented=on
  drive pulley velocity : Outport
  load velocity : Outport  Port=2
  load position : Outport  Port=3
  driven pulley Velocity : Outport  Port=4
  wires:
  Gain23/1 -> Minus2/3
  Gain4/1 -> Gain5/1
  [theta1] -> Gain24/1
  Gain11/1 -> Minus1/1
  [theta3_dot] -> Gain26/1
  Gain26/1 -> Minus2/5
  Gain22/1 -> Gain23/1
  Gain19/1 -> Minus2/1
  Gain21/1 -> Minus2/2
  Integrator/1 -> Integrator1/1, [theta1_dot], Gain8/1  "theta1_dot"
  Integrator1/1 -> Gain6/1, Gain2/1, [theta1]  "theta1"
  Integrator6/1 -> Integrator7/1, [x2_dot]  "x2_dot"
  Gain3/1 -> Minus/3
  Gain18/1 -> Gain19/1
  Gain1/1 -> Minus/4
  Gain2/1 -> Gain3/1
  Integrator2/1 -> [theta3_dot], Integrator4/1  "theta3_dot"
  Integrator4/1 -> Gain4/1, [theta3]  "theta3"
  [x2] -> Gain12/1
  Gain/1 -> Gain1/1
  Gain10/1 -> Gain11/1
  Gain24/1 -> Gain25/1
  Gain13/1 -> Minus1/3
  [theta3] -> Gain20/1
  [theta3] -> Gain14/1
  Gain15/1 -> Minus1/4
  Gain6/1 -> Gain7/1
  [theta3] -> Gain22/1
  Gain5/1 -> Minus/5
  [theta1] -> Gain10/1
  [x2] -> Gain18/1
  Minus2/1 -> Gain27/1
  Minus1/1 -> Gain17/1
  Minus/1 -> Gain9/1
  Gain7/1 -> Minus/2
  Integrator7/1 -> Gain/1, [x2]  "x2"
  Gain16/1 -> Minus1/5
  Gain8/1 -> Minus/1
  Gain17/1 -> Integrator6/1  "x2_dot_dot"
  Gain14/1 -> Gain15/1
  Gain20/1 -> Gain21/1
  Gain9/1 -> Integrator/1  "theta1_dot_dot"
  Gain12/1 -> Minus1/2
  Gain25/1 -> Minus2/4
  [x2] -> Gain13/1
  [x2_dot] -> Gain16/1
  [theta1_dot] -> drive pulley velocity/1
  [x2_dot] -> load velocity/1
  Gain27/1 -> Integrator2/1  "theta3_dot_dot"
  DC Motor1/1(Tourque) -> Minus/6  "Tourque"
  [x2_dot] -> DC Motor1/2(Velocity)
  Voltage/1 -> DC Motor1/1(Voltage)
  [x2] -> load position/1
  [theta3_dot] -> driven pulley Velocity/1

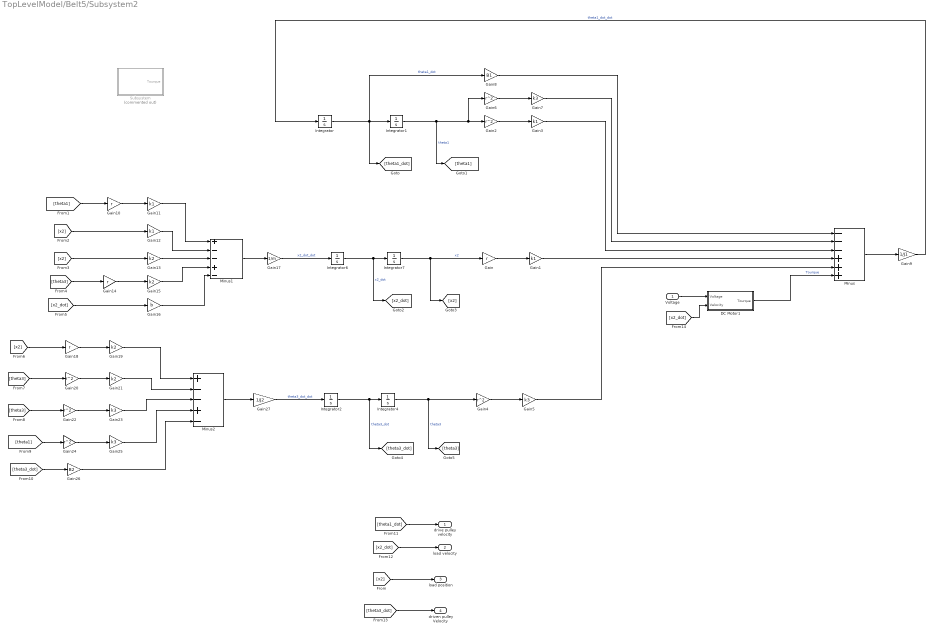
== system TopLevelModel/Belt5/Subsystem2 ==
  Voltage : Inport
  DC Motor1 : Subsystem
  Gain{,10,14,18} (4 alike) : Gain  Gain=r
  Gain{1,3,11..12} (4 alike) : Gain  Gain=k1
  Gain{13,15,19,21} (4 alike) : Gain  Gain=k2
  Gain16 : Gain  Gain=b
  Gain17 : Gain  Gain=1/m
  Gain{2,4,6,20,22,24} (6 alike) : Gain  Gain=r^2
  Gain{5,7,23,25} (4 alike) : Gain  Gain=k3
  Gain26 : Gain  Gain=B2
  Gain27 : Gain  Gain=1/J2
  Gain8 : Gain  Gain=B1
  Gain9 : Gain  Gain=1/J1
  Integrator{,1..2,4,6..7} (6 alike) : Integrator
  Minus : Sum  Inputs=---+++
  Minus1 : Sum  Inputs=+--+-
  Minus2 : Sum  Inputs=+--+-
  Subsystem : Subsystem  Commented=on
  drive pulley velocity : Outport
  load velocity : Outport  Port=2
  load position : Outport  Port=3
  driven pulley Velocity : Outport  Port=4
  wires:
  Gain23/1 -> Minus2/3
  Gain4/1 -> Gain5/1
  [theta1] -> Gain24/1
  Gain11/1 -> Minus1/1
  [theta3_dot] -> Gain26/1
  Gain26/1 -> Minus2/5
  Gain22/1 -> Gain23/1
  Gain19/1 -> Minus2/1
  Gain21/1 -> Minus2/2
  Integrator/1 -> Integrator1/1, [theta1_dot], Gain8/1  "theta1_dot"
  Integrator1/1 -> Gain6/1, Gain2/1, [theta1]  "theta1"
  Integrator6/1 -> Integrator7/1, [x2_dot]  "x2_dot"
  Gain3/1 -> Minus/3
  Gain18/1 -> Gain19/1
  Gain1/1 -> Minus/4
  Gain2/1 -> Gain3/1
  Integrator2/1 -> [theta3_dot], Integrator4/1  "theta3_dot"
  Integrator4/1 -> Gain4/1, [theta3]  "theta3"
  [x2] -> Gain12/1
  Gain/1 -> Gain1/1
  Gain10/1 -> Gain11/1
  Gain24/1 -> Gain25/1
  Gain13/1 -> Minus1/3
  [theta3] -> Gain20/1
  [theta3] -> Gain14/1
  Gain15/1 -> Minus1/4
  Gain6/1 -> Gain7/1
  [theta3] -> Gain22/1
  Gain5/1 -> Minus/5
  [theta1] -> Gain10/1
  [x2] -> Gain18/1
  Minus2/1 -> Gain27/1
  Minus1/1 -> Gain17/1
  Minus/1 -> Gain9/1
  Gain7/1 -> Minus/2
  Integrator7/1 -> Gain/1, [x2]  "x2"
  Gain16/1 -> Minus1/5
  Gain8/1 -> Minus/1
  Gain17/1 -> Integrator6/1  "x2_dot_dot"
  Gain14/1 -> Gain15/1
  Gain20/1 -> Gain21/1
  Gain9/1 -> Integrator/1  "theta1_dot_dot"
  Gain12/1 -> Minus1/2
  Gain25/1 -> Minus2/4
  [x2] -> Gain13/1
  [x2_dot] -> Gain16/1
  [theta1_dot] -> drive pulley velocity/1
  [x2_dot] -> load velocity/1
  Gain27/1 -> Integrator2/1  "theta3_dot_dot"
  DC Motor1/1(Tourque) -> Minus/6  "Tourque"
  [x2_dot] -> DC Motor1/2(Velocity)
  Voltage/1 -> DC Motor1/1(Voltage)
  [x2] -> load position/1
  [theta3_dot] -> driven pulley Velocity/1

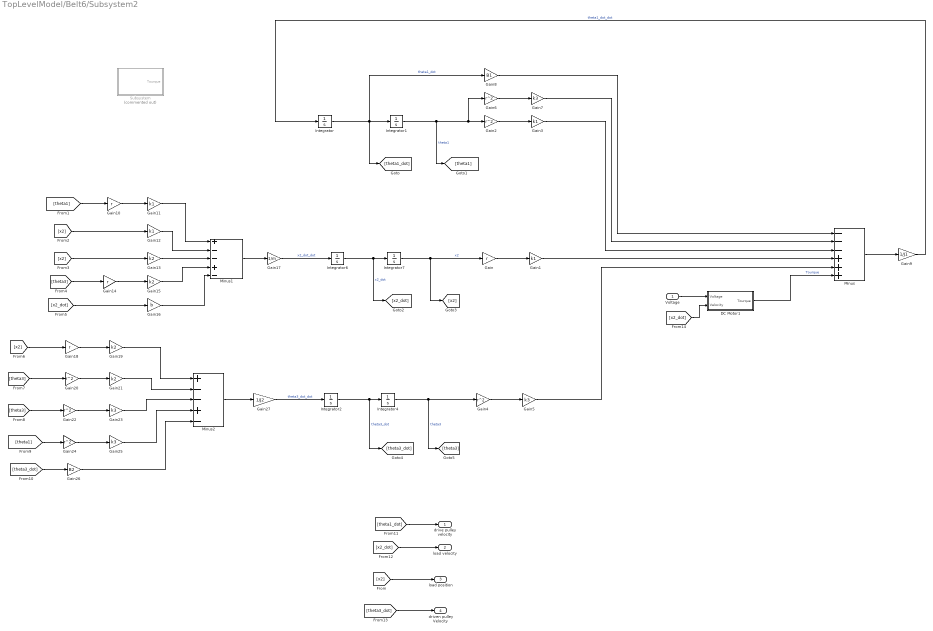
== system TopLevelModel/Belt6/Subsystem2 ==
  Voltage : Inport
  DC Motor1 : Subsystem
  Gain{,10,14,18} (4 alike) : Gain  Gain=r
  Gain{1,3,11..12} (4 alike) : Gain  Gain=k1
  Gain{13,15,19,21} (4 alike) : Gain  Gain=k2
  Gain16 : Gain  Gain=b
  Gain17 : Gain  Gain=1/m
  Gain{2,4,6,20,22,24} (6 alike) : Gain  Gain=r^2
  Gain{5,7,23,25} (4 alike) : Gain  Gain=k3
  Gain26 : Gain  Gain=B2
  Gain27 : Gain  Gain=1/J2
  Gain8 : Gain  Gain=B1
  Gain9 : Gain  Gain=1/J1
  Integrator{,1..2,4,6..7} (6 alike) : Integrator
  Minus : Sum  Inputs=---+++
  Minus1 : Sum  Inputs=+--+-
  Minus2 : Sum  Inputs=+--+-
  Subsystem : Subsystem  Commented=on
  drive pulley velocity : Outport
  load velocity : Outport  Port=2
  load position : Outport  Port=3
  driven pulley Velocity : Outport  Port=4
  wires:
  Gain23/1 -> Minus2/3
  Gain4/1 -> Gain5/1
  [theta1] -> Gain24/1
  Gain11/1 -> Minus1/1
  [theta3_dot] -> Gain26/1
  Gain26/1 -> Minus2/5
  Gain22/1 -> Gain23/1
  Gain19/1 -> Minus2/1
  Gain21/1 -> Minus2/2
  Integrator/1 -> Integrator1/1, [theta1_dot], Gain8/1  "theta1_dot"
  Integrator1/1 -> Gain6/1, Gain2/1, [theta1]  "theta1"
  Integrator6/1 -> Integrator7/1, [x2_dot]  "x2_dot"
  Gain3/1 -> Minus/3
  Gain18/1 -> Gain19/1
  Gain1/1 -> Minus/4
  Gain2/1 -> Gain3/1
  Integrator2/1 -> [theta3_dot], Integrator4/1  "theta3_dot"
  Integrator4/1 -> Gain4/1, [theta3]  "theta3"
  [x2] -> Gain12/1
  Gain/1 -> Gain1/1
  Gain10/1 -> Gain11/1
  Gain24/1 -> Gain25/1
  Gain13/1 -> Minus1/3
  [theta3] -> Gain20/1
  [theta3] -> Gain14/1
  Gain15/1 -> Minus1/4
  Gain6/1 -> Gain7/1
  [theta3] -> Gain22/1
  Gain5/1 -> Minus/5
  [theta1] -> Gain10/1
  [x2] -> Gain18/1
  Minus2/1 -> Gain27/1
  Minus1/1 -> Gain17/1
  Minus/1 -> Gain9/1
  Gain7/1 -> Minus/2
  Integrator7/1 -> Gain/1, [x2]  "x2"
  Gain16/1 -> Minus1/5
  Gain8/1 -> Minus/1
  Gain17/1 -> Integrator6/1  "x2_dot_dot"
  Gain14/1 -> Gain15/1
  Gain20/1 -> Gain21/1
  Gain9/1 -> Integrator/1  "theta1_dot_dot"
  Gain12/1 -> Minus1/2
  Gain25/1 -> Minus2/4
  [x2] -> Gain13/1
  [x2_dot] -> Gain16/1
  [theta1_dot] -> drive pulley velocity/1
  [x2_dot] -> load velocity/1
  Gain27/1 -> Integrator2/1  "theta3_dot_dot"
  DC Motor1/1(Tourque) -> Minus/6  "Tourque"
  [x2_dot] -> DC Motor1/2(Velocity)
  Voltage/1 -> DC Motor1/1(Voltage)
  [x2] -> load position/1
  [theta3_dot] -> driven pulley Velocity/1

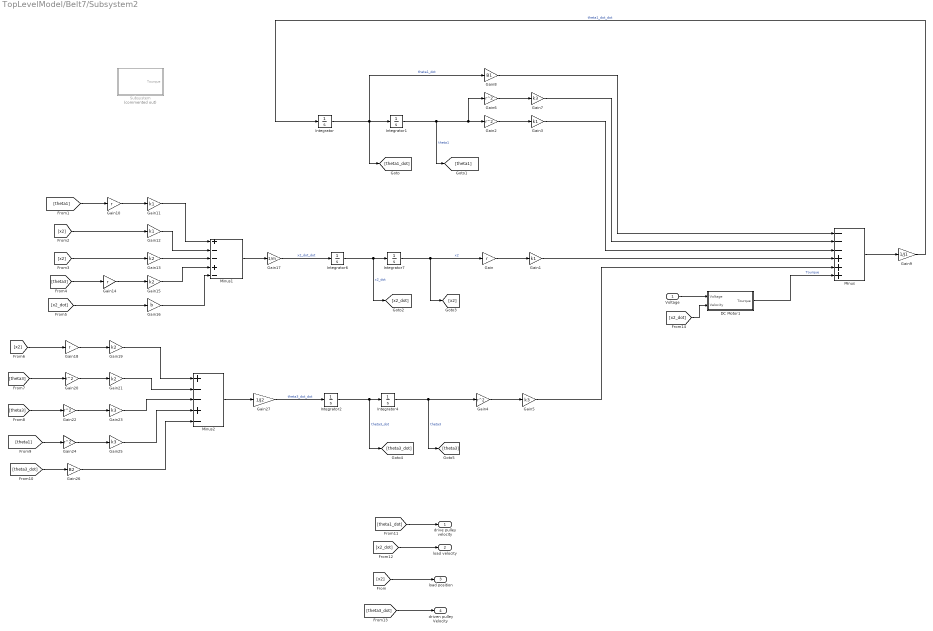
== system TopLevelModel/Belt7/Subsystem2 ==
  Voltage : Inport
  DC Motor1 : Subsystem
  Gain{,10,14,18} (4 alike) : Gain  Gain=r
  Gain{1,3,11..12} (4 alike) : Gain  Gain=k1
  Gain{13,15,19,21} (4 alike) : Gain  Gain=k2
  Gain16 : Gain  Gain=b
  Gain17 : Gain  Gain=1/m
  Gain{2,4,6,20,22,24} (6 alike) : Gain  Gain=r^2
  Gain{5,7,23,25} (4 alike) : Gain  Gain=k3
  Gain26 : Gain  Gain=B2
  Gain27 : Gain  Gain=1/J2
  Gain8 : Gain  Gain=B1
  Gain9 : Gain  Gain=1/J1
  Integrator{,1..2,4,6..7} (6 alike) : Integrator
  Minus : Sum  Inputs=---+++
  Minus1 : Sum  Inputs=+--+-
  Minus2 : Sum  Inputs=+--+-
  Subsystem : Subsystem  Commented=on
  drive pulley velocity : Outport
  load velocity : Outport  Port=2
  load position : Outport  Port=3
  driven pulley Velocity : Outport  Port=4
  wires:
  Gain23/1 -> Minus2/3
  Gain4/1 -> Gain5/1
  [theta1] -> Gain24/1
  Gain11/1 -> Minus1/1
  [theta3_dot] -> Gain26/1
  Gain26/1 -> Minus2/5
  Gain22/1 -> Gain23/1
  Gain19/1 -> Minus2/1
  Gain21/1 -> Minus2/2
  Integrator/1 -> Integrator1/1, [theta1_dot], Gain8/1  "theta1_dot"
  Integrator1/1 -> Gain6/1, Gain2/1, [theta1]  "theta1"
  Integrator6/1 -> Integrator7/1, [x2_dot]  "x2_dot"
  Gain3/1 -> Minus/3
  Gain18/1 -> Gain19/1
  Gain1/1 -> Minus/4
  Gain2/1 -> Gain3/1
  Integrator2/1 -> [theta3_dot], Integrator4/1  "theta3_dot"
  Integrator4/1 -> Gain4/1, [theta3]  "theta3"
  [x2] -> Gain12/1
  Gain/1 -> Gain1/1
  Gain10/1 -> Gain11/1
  Gain24/1 -> Gain25/1
  Gain13/1 -> Minus1/3
  [theta3] -> Gain20/1
  [theta3] -> Gain14/1
  Gain15/1 -> Minus1/4
  Gain6/1 -> Gain7/1
  [theta3] -> Gain22/1
  Gain5/1 -> Minus/5
  [theta1] -> Gain10/1
  [x2] -> Gain18/1
  Minus2/1 -> Gain27/1
  Minus1/1 -> Gain17/1
  Minus/1 -> Gain9/1
  Gain7/1 -> Minus/2
  Integrator7/1 -> Gain/1, [x2]  "x2"
  Gain16/1 -> Minus1/5
  Gain8/1 -> Minus/1
  Gain17/1 -> Integrator6/1  "x2_dot_dot"
  Gain14/1 -> Gain15/1
  Gain20/1 -> Gain21/1
  Gain9/1 -> Integrator/1  "theta1_dot_dot"
  Gain12/1 -> Minus1/2
  Gain25/1 -> Minus2/4
  [x2] -> Gain13/1
  [x2_dot] -> Gain16/1
  [theta1_dot] -> drive pulley velocity/1
  [x2_dot] -> load velocity/1
  Gain27/1 -> Integrator2/1  "theta3_dot_dot"
  DC Motor1/1(Tourque) -> Minus/6  "Tourque"
  [x2_dot] -> DC Motor1/2(Velocity)
  Voltage/1 -> DC Motor1/1(Voltage)
  [x2] -> load position/1
  [theta3_dot] -> driven pulley Velocity/1

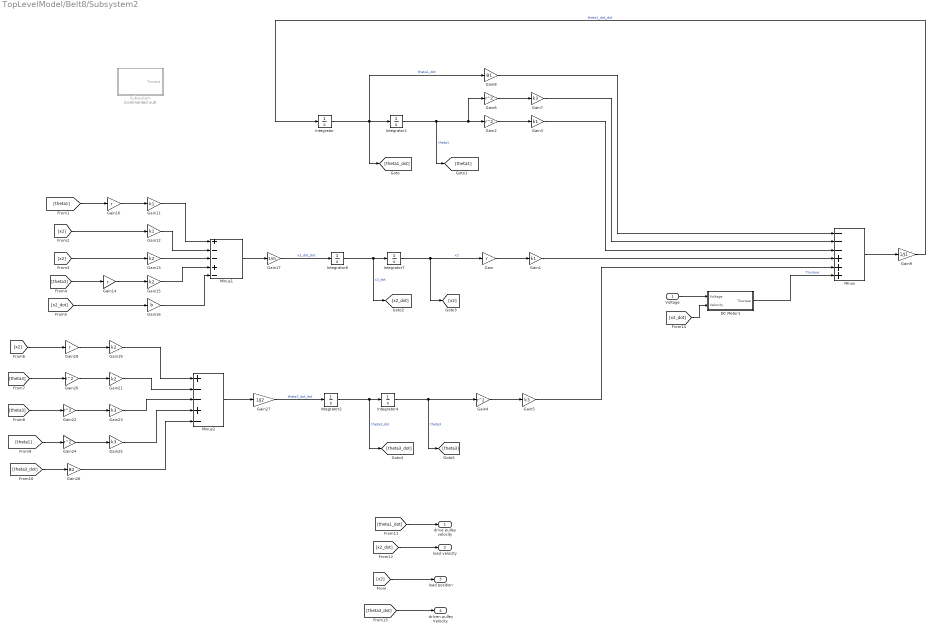
== system TopLevelModel/Belt8/Subsystem2 ==
  Voltage : Inport
  DC Motor1 : Subsystem
  Gain{,10,14,18} (4 alike) : Gain  Gain=r
  Gain{1,3,11..12} (4 alike) : Gain  Gain=k1
  Gain{13,15,19,21} (4 alike) : Gain  Gain=k2
  Gain16 : Gain  Gain=b
  Gain17 : Gain  Gain=1/m
  Gain{2,4,6,20,22,24} (6 alike) : Gain  Gain=r^2
  Gain{5,7,23,25} (4 alike) : Gain  Gain=k3
  Gain26 : Gain  Gain=B2
  Gain27 : Gain  Gain=1/J2
  Gain8 : Gain  Gain=B1
  Gain9 : Gain  Gain=1/J1
  Integrator{,1..2,4,6..7} (6 alike) : Integrator
  Minus : Sum  Inputs=---+++
  Minus1 : Sum  Inputs=+--+-
  Minus2 : Sum  Inputs=+--+-
  Subsystem : Subsystem  Commented=on
  drive pulley velocity : Outport
  load velocity : Outport  Port=2
  load position : Outport  Port=3
  driven pulley Velocity : Outport  Port=4
  wires:
  Gain23/1 -> Minus2/3
  Gain4/1 -> Gain5/1
  [theta1] -> Gain24/1
  Gain11/1 -> Minus1/1
  [theta3_dot] -> Gain26/1
  Gain26/1 -> Minus2/5
  Gain22/1 -> Gain23/1
  Gain19/1 -> Minus2/1
  Gain21/1 -> Minus2/2
  Integrator/1 -> Integrator1/1, [theta1_dot], Gain8/1  "theta1_dot"
  Integrator1/1 -> Gain6/1, Gain2/1, [theta1]  "theta1"
  Integrator6/1 -> Integrator7/1, [x2_dot]  "x2_dot"
  Gain3/1 -> Minus/3
  Gain18/1 -> Gain19/1
  Gain1/1 -> Minus/4
  Gain2/1 -> Gain3/1
  Integrator2/1 -> [theta3_dot], Integrator4/1  "theta3_dot"
  Integrator4/1 -> Gain4/1, [theta3]  "theta3"
  [x2] -> Gain12/1
  Gain/1 -> Gain1/1
  Gain10/1 -> Gain11/1
  Gain24/1 -> Gain25/1
  Gain13/1 -> Minus1/3
  [theta3] -> Gain20/1
  [theta3] -> Gain14/1
  Gain15/1 -> Minus1/4
  Gain6/1 -> Gain7/1
  [theta3] -> Gain22/1
  Gain5/1 -> Minus/5
  [theta1] -> Gain10/1
  [x2] -> Gain18/1
  Minus2/1 -> Gain27/1
  Minus1/1 -> Gain17/1
  Minus/1 -> Gain9/1
  Gain7/1 -> Minus/2
  Integrator7/1 -> Gain/1, [x2]  "x2"
  Gain16/1 -> Minus1/5
  Gain8/1 -> Minus/1
  Gain17/1 -> Integrator6/1  "x2_dot_dot"
  Gain14/1 -> Gain15/1
  Gain20/1 -> Gain21/1
  Gain9/1 -> Integrator/1  "theta1_dot_dot"
  Gain12/1 -> Minus1/2
  Gain25/1 -> Minus2/4
  [x2] -> Gain13/1
  [x2_dot] -> Gain16/1
  [theta1_dot] -> drive pulley velocity/1
  [x2_dot] -> load velocity/1
  Gain27/1 -> Integrator2/1  "theta3_dot_dot"
  DC Motor1/1(Tourque) -> Minus/6  "Tourque"
  [x2_dot] -> DC Motor1/2(Velocity)
  Voltage/1 -> DC Motor1/1(Voltage)
  [x2] -> load position/1
  [theta3_dot] -> driven pulley Velocity/1

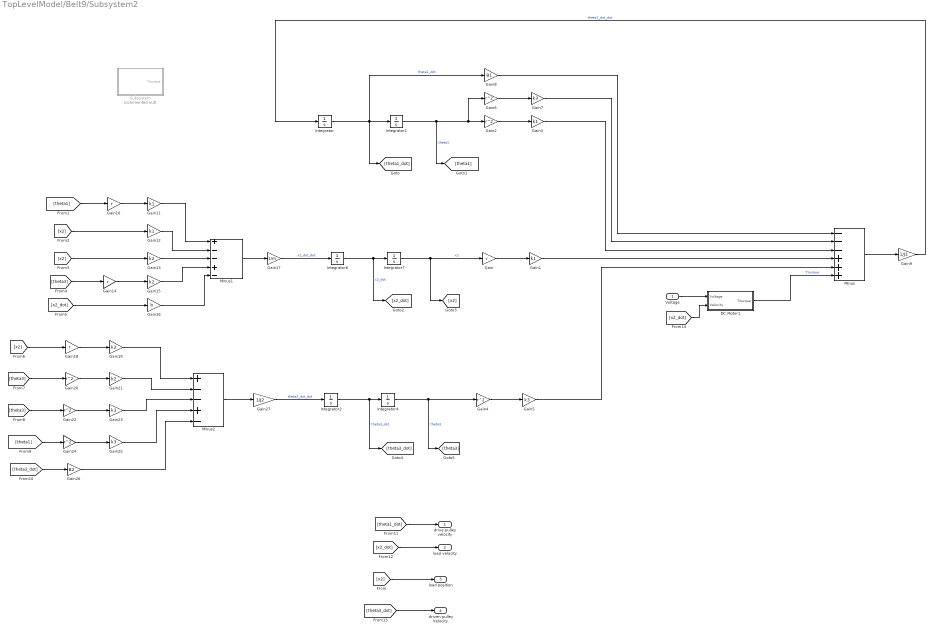
== system TopLevelModel/Belt9/Subsystem2 ==
  Voltage : Inport
  DC Motor1 : Subsystem
  Gain{,10,14,18} (4 alike) : Gain  Gain=r
  Gain{1,3,11..12} (4 alike) : Gain  Gain=k1
  Gain{13,15,19,21} (4 alike) : Gain  Gain=k2
  Gain16 : Gain  Gain=b
  Gain17 : Gain  Gain=1/m
  Gain{2,4,6,20,22,24} (6 alike) : Gain  Gain=r^2
  Gain{5,7,23,25} (4 alike) : Gain  Gain=k3
  Gain26 : Gain  Gain=B2
  Gain27 : Gain  Gain=1/J2
  Gain8 : Gain  Gain=B1
  Gain9 : Gain  Gain=1/J1
  Integrator{,1..2,4,6..7} (6 alike) : Integrator
  Minus : Sum  Inputs=---+++
  Minus1 : Sum  Inputs=+--+-
  Minus2 : Sum  Inputs=+--+-
  Subsystem : Subsystem  Commented=on
  drive pulley velocity : Outport
  load velocity : Outport  Port=2
  load position : Outport  Port=3
  driven pulley Velocity : Outport  Port=4
  wires:
  Gain23/1 -> Minus2/3
  Gain4/1 -> Gain5/1
  [theta1] -> Gain24/1
  Gain11/1 -> Minus1/1
  [theta3_dot] -> Gain26/1
  Gain26/1 -> Minus2/5
  Gain22/1 -> Gain23/1
  Gain19/1 -> Minus2/1
  Gain21/1 -> Minus2/2
  Integrator/1 -> Integrator1/1, [theta1_dot], Gain8/1  "theta1_dot"
  Integrator1/1 -> Gain6/1, Gain2/1, [theta1]  "theta1"
  Integrator6/1 -> Integrator7/1, [x2_dot]  "x2_dot"
  Gain3/1 -> Minus/3
  Gain18/1 -> Gain19/1
  Gain1/1 -> Minus/4
  Gain2/1 -> Gain3/1
  Integrator2/1 -> [theta3_dot], Integrator4/1  "theta3_dot"
  Integrator4/1 -> Gain4/1, [theta3]  "theta3"
  [x2] -> Gain12/1
  Gain/1 -> Gain1/1
  Gain10/1 -> Gain11/1
  Gain24/1 -> Gain25/1
  Gain13/1 -> Minus1/3
  [theta3] -> Gain20/1
  [theta3] -> Gain14/1
  Gain15/1 -> Minus1/4
  Gain6/1 -> Gain7/1
  [theta3] -> Gain22/1
  Gain5/1 -> Minus/5
  [theta1] -> Gain10/1
  [x2] -> Gain18/1
  Minus2/1 -> Gain27/1
  Minus1/1 -> Gain17/1
  Minus/1 -> Gain9/1
  Gain7/1 -> Minus/2
  Integrator7/1 -> Gain/1, [x2]  "x2"
  Gain16/1 -> Minus1/5
  Gain8/1 -> Minus/1
  Gain17/1 -> Integrator6/1  "x2_dot_dot"
  Gain14/1 -> Gain15/1
  Gain20/1 -> Gain21/1
  Gain9/1 -> Integrator/1  "theta1_dot_dot"
  Gain12/1 -> Minus1/2
  Gain25/1 -> Minus2/4
  [x2] -> Gain13/1
  [x2_dot] -> Gain16/1
  [theta1_dot] -> drive pulley velocity/1
  [x2_dot] -> load velocity/1
  Gain27/1 -> Integrator2/1  "theta3_dot_dot"
  DC Motor1/1(Tourque) -> Minus/6  "Tourque"
  [x2_dot] -> DC Motor1/2(Velocity)
  Voltage/1 -> DC Motor1/1(Voltage)
  [x2] -> load position/1
  [theta3_dot] -> driven pulley Velocity/1

== system TopLevelModel/Controller/Position ==
  Ref : Inport
  Algorithm and Pulse Generation : Subsystem
  ERef : fl_lib/Electrical/Electrical Elements/Electrical Reference
  PWM : PMIOPort  Side=Right
  0v : PMIOPort  Port=2  Side=Right
  REV : PMIOPort  Port=3  Side=Right
  wires:
  Ref/1 -> Algorithm and Pulse Generation/1(Reference)
  connections:
  Algorithm and Pulse Generation/RConn2 -- PWM/RConn1
  Algorithm and Pulse Generation/RConn1 -- REV/RConn1
  ERef/LConn1 -- 0v/RConn1

== system TopLevelModel/Controller/Speed ==
  note: Step rate and direction algorithm implemented on a microprocessor or dedicated discrete chip
  Ref : Inport
  ERef : fl_lib/Electrical/Electrical Elements/Electrical Reference
  Step Rate and Direction : Subsystem
  Voltage-Controlled Pulse Generator : Subsystem
  PWM : PMIOPort  Side=Right
  0v : PMIOPort  Port=2  Side=Right
  REV : PMIOPort  Port=3  Side=Right
  wires:
  Ref/1 -> Step Rate and Direction/1(Reference)
  connections:
  PWM/RConn1 -- Voltage-Controlled Pulse Generator/RConn1
  Voltage-Controlled Pulse Generator/RConn2 -- 0v/RConn1 -- ERef/LConn1
  Step Rate and Direction/RConn1 -- REV/RConn1
  Step Rate and Direction/RConn2 -- Voltage-Controlled Pulse Generator/LConn1

== system TopLevelModel/Controller1/Position ==
  Ref : Inport
  Algorithm and Pulse Generation : Subsystem
  ERef : fl_lib/Electrical/Electrical Elements/Electrical Reference
  PWM : PMIOPort  Side=Right
  0v : PMIOPort  Port=2  Side=Right
  REV : PMIOPort  Port=3  Side=Right
  wires:
  Ref/1 -> Algorithm and Pulse Generation/1(Reference)
  connections:
  Algorithm and Pulse Generation/RConn2 -- PWM/RConn1
  Algorithm and Pulse Generation/RConn1 -- REV/RConn1
  ERef/LConn1 -- 0v/RConn1

== system TopLevelModel/Controller1/Speed ==
  note: Step rate and direction algorithm implemented on a microprocessor or dedicated discrete chip
  Ref : Inport
  ERef : fl_lib/Electrical/Electrical Elements/Electrical Reference
  Step Rate and Direction : Subsystem
  Voltage-Controlled Pulse Generator : Subsystem
  PWM : PMIOPort  Side=Right
  0v : PMIOPort  Port=2  Side=Right
  REV : PMIOPort  Port=3  Side=Right
  wires:
  Ref/1 -> Step Rate and Direction/1(Reference)
  connections:
  PWM/RConn1 -- Voltage-Controlled Pulse Generator/RConn1
  Voltage-Controlled Pulse Generator/RConn2 -- 0v/RConn1 -- ERef/LConn1
  Step Rate and Direction/RConn1 -- REV/RConn1
  Step Rate and Direction/RConn2 -- Voltage-Controlled Pulse Generator/LConn1

== system TopLevelModel/Subsystem/DC Motor1 ==
  note: Armature Controlled DC Motor
      |
      | $E_a = R_a \cdot I_a + L_a \cdot \frac{di_a}{dt} + K_b \cdot \frac{d\theta}{dt}$
      | $T_{m} = K_{t} \cdot I_{a}$
  Voltage : Inport
  Velocity : Inport  Port=2
  Constant1 : Constant  Value=R
  Gain1 : Gain  Gain=Kb
  Gain2 : Gain  Gain=1/L
  Gain3 : Gain  Gain=Kt
  Integrator : Integrator
  Product : Product
  Subtract : Sum  Inputs=+--
  Tourque : Outport
  wires:
  Voltage/1 -> Subtract/1
  Integrator/1 -> Product/1, Gain3/1  "i"
  Gain3/1 -> Tourque/1
  Gain1/1 -> Subtract/2
  Velocity/1 -> Gain1/1
  Constant1/1 -> Product/2
  Product/1 -> Subtract/3
  Gain2/1 -> Integrator/1  "i_dot"
  Subtract/1 -> Gain2/1

== system TopLevelModel/Subsystem1/DC Motor1 ==
  note: Armature Controlled DC Motor
      |
      | $E_a = R_a \cdot I_a + L_a \cdot \frac{di_a}{dt} + K_b \cdot \frac{d\theta}{dt}$
      | $T_{m} = K_{t} \cdot I_{a}$
  Voltage : Inport
  Velocity : Inport  Port=2
  Constant1 : Constant  Value=R
  Gain1 : Gain  Gain=Kb
  Gain2 : Gain  Gain=1/L
  Gain3 : Gain  Gain=Kt
  Integrator : Integrator
  Product : Product
  Subtract : Sum  Inputs=+--
  Tourque : Outport
  wires:
  Voltage/1 -> Subtract/1
  Integrator/1 -> Product/1, Gain3/1  "i"
  Gain3/1 -> Tourque/1
  Gain1/1 -> Subtract/2
  Velocity/1 -> Gain1/1
  Constant1/1 -> Product/2
  Product/1 -> Subtract/3
  Gain2/1 -> Integrator/1  "i_dot"
  Subtract/1 -> Gain2/1

== system TopLevelModel/Subsystem1/Subsystem ==
  Constant : Constant  Value=Kt
  Constant1 : Constant  Value=Ke
  Constant2 : Constant  Value=R
  Divide : Product  Inputs=**/
  Divide1 : Product  Inputs=***/
  Minus3 : Sum  Inputs=+-
  Voltage : DiscretePulseGenerator  PulseType=Time based  Amplitude=12  Period=11  PulseWidth=50  PhaseDelay=2
  Tourque : Outport
  wires:
  Divide1/1 -> Minus3/2
  Divide/1 -> Minus3/1
  Constant/1 -> Divide/2, Divide1/1
  [theta1_dot] -> Divide1/3
  Constant1/1 -> Divide1/2
  Constant2/1 -> Divide1/4, Divide/3
  Minus3/1 -> Tourque/1  "Tourque"
  Voltage/1 -> Divide/1

== system TopLevelModel/Belt1/Subsystem2/DC Motor1 ==
  note: Armature Controlled DC Motor
      |
      | $E_a = R_a \cdot I_a + L_a \cdot \frac{di_a}{dt} + K_b \cdot \frac{d\theta}{dt}$
      | $T_{m} = K_{t} \cdot I_{a}$
  Voltage : Inport
  Velocity : Inport  Port=2
  Constant1 : Constant  Value=R
  Gain1 : Gain  Gain=Kb
  Gain2 : Gain  Gain=1/L
  Gain3 : Gain  Gain=Kt
  Integrator : Integrator
  Product : Product
  Subtract : Sum  Inputs=+--
  Tourque : Outport
  wires:
  Voltage/1 -> Subtract/1
  Integrator/1 -> Product/1, Gain3/1  "i"
  Gain3/1 -> Tourque/1
  Gain1/1 -> Subtract/2
  Velocity/1 -> Gain1/1
  Constant1/1 -> Product/2
  Product/1 -> Subtract/3
  Gain2/1 -> Integrator/1  "i_dot"
  Subtract/1 -> Gain2/1

== system TopLevelModel/Belt1/Subsystem2/Subsystem ==
  Constant : Constant  Value=Kt
  Constant1 : Constant  Value=Ke
  Constant2 : Constant  Value=R
  Divide : Product  Inputs=**/
  Divide1 : Product  Inputs=***/
  Minus3 : Sum  Inputs=+-
  Voltage : DiscretePulseGenerator  PulseType=Time based  Amplitude=12  Period=11  PulseWidth=50  PhaseDelay=2
  Tourque : Outport
  wires:
  Divide1/1 -> Minus3/2
  Divide/1 -> Minus3/1
  Constant/1 -> Divide/2, Divide1/1
  [theta1_dot] -> Divide1/3
  Constant1/1 -> Divide1/2
  Constant2/1 -> Divide1/4, Divide/3
  Minus3/1 -> Tourque/1  "Tourque"
  Voltage/1 -> Divide/1

== system TopLevelModel/Belt2/Subsystem2/DC Motor1 ==
  note: Armature Controlled DC Motor
      |
      | $E_a = R_a \cdot I_a + L_a \cdot \frac{di_a}{dt} + K_b \cdot \frac{d\theta}{dt}$
      | $T_{m} = K_{t} \cdot I_{a}$
  Voltage : Inport
  Velocity : Inport  Port=2
  Constant1 : Constant  Value=R
  Gain1 : Gain  Gain=Kb
  Gain2 : Gain  Gain=1/L
  Gain3 : Gain  Gain=Kt
  Integrator : Integrator
  Product : Product
  Subtract : Sum  Inputs=+--
  Tourque : Outport
  wires:
  Voltage/1 -> Subtract/1
  Integrator/1 -> Product/1, Gain3/1  "i"
  Gain3/1 -> Tourque/1
  Gain1/1 -> Subtract/2
  Velocity/1 -> Gain1/1
  Constant1/1 -> Product/2
  Product/1 -> Subtract/3
  Gain2/1 -> Integrator/1  "i_dot"
  Subtract/1 -> Gain2/1
